simulink model "SCARA_Ass5_Script_Visual"  (Simulink 7.4)
settings: Solver=FixedStepDiscrete  StartTime=0.0  StopTime=inf  FixedStep=0.00001  RelTol=1e-3
libraries: vrlib x1
settings Model: Creator=Mengchen  LastModifiedBy=t6z8
settings OptimizationCC: ExpressionDepthLimit=128  InitFltsAndDblsToZero=on
settings DebuggingCC: AlgebraicLoopMsg=error  SaveWithParameterizedLinksMsg=none  StateNameClashWarn=none  StrictBusMsg=ErrorLevel1
settings HardwareCC: TargetEndianess=LittleEndian  TargetHWDeviceType=MATLAB Host
settings RTWCC: ProcessScript=grt_make_rtw_hook  CustomHeaderCode="#include \"haptics.h\""  CustomInclude="\"C:\\Program Files\\novint\\HDAL_SDK_1.1.0_Beta\\include\""  TargetLang=C++
settings CodeAppCC: CustomSymbolStrType=$N$R$M_T

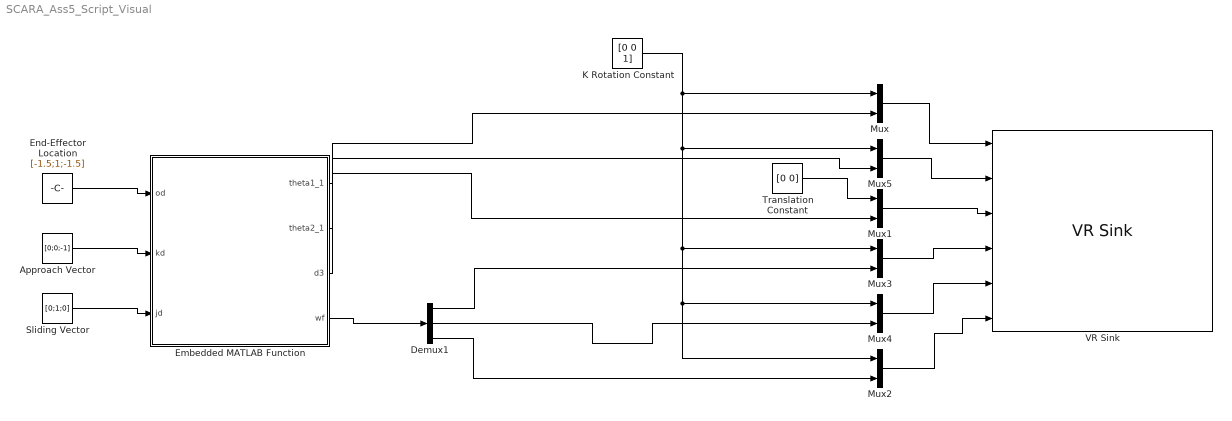
== system SCARA_Ass5_Script_Visual ==
  Approach Vector : Constant  Value=[0;0;-1]
  Demux1 : Demux  Outputs=3
  Embedded MATLAB Function : Stateflow chart
  End-Effector Location : Constant  Value=[-1.5;1;-1.5]
  K Rotation Constant : Constant  Value=[0 0 1]
  Mux{,1..5} (6 alike) : Mux  Inputs=2
  Sliding Vector : Constant  Value=[0;1;0]
  Translation Constant : Constant  Value=[0 0]
  VR Sink : vrlib/VR Sink  InstantiateOnLoad=on  SampleTime=-1  ViewEnable=on  RemoteChange=off  RemoteView=on  FieldsWritten=Link_0_Rotation.rotation.4.1.double#Link_1_Rotation.rotation.4.1.double#Link_2_Translation.translation.3.1.double#Link_3_Rotation.rotation.4.1.double#Link_4_Rotation.rotation.4.1.double#Link_5_Rotation.rotation.4.1.double  WorldFileName=SCARAWORLD.WRL  AutoView=off  VideoDimensions=[]  FigureProperties="{'Position', 'Name', 'Viewpoint', 'CameraBound', 'CameraDirection', 'CameraPosition', 'CameraUpVector', 'ZoomFactor', 'Antialiasing', 'Headlight', 'Lighting', 'NavPanel', 'StatusBar', 'ToolBar', 'Textures', 'Transparency', 'Wireframe', 'NavZones', 'NavMode', 'NavSpeed', 'Record2DCompressMethod', 'Record2DCompressQuality', 'Record2D', 'Record2DFileName', 'Record2DFPS'; [7.7000000000000000e+002  2.2200000000000000e+002  5.7600000000000000e+002  3.8000000000000000e+002], '', 'Viewpoint', 'on', [0.0000000000000000e+000  0.0000000000000000e+000 -1.0000000000000000e+000], [0.0000000000000000e+000  0.0000000000000000e+000  0.0000000000000000e+000], [0.0000000000000000e+000  1.0000000000000000e+000  0.0000000000000000e+000], [1.0000000000000000e+000], 'off', 'on', 'on', 'halfbar', 'on', 'on', 'on', 'on', 'off', 'off', 'fly', 'normal', 'auto', [7.5000000000000000e+001], 'off', '%f_anim_%n.avi', [1.5000000000000000e+001]}"
  wires:
  K Rotation Constant/1 -> Mux/1, Mux3/1, Mux4/1, Mux2/1, Mux5/1
  Mux/1 -> VR Sink/1
  Mux1/1 -> VR Sink/3
  Translation Constant/1 -> Mux1/1
  Mux3/1 -> VR Sink/4
  Mux4/1 -> VR Sink/5
  Mux2/1 -> VR Sink/6
  Mux5/1 -> VR Sink/2
  Embedded MATLAB Function/1(theta1_1) -> Mux/2
  Embedded MATLAB Function/2(theta2_1) -> Mux5/2
  Embedded MATLAB Function/3(d3) -> Mux1/2
  Demux1/1 -> Mux3/2
  Demux1/2 -> Mux4/2
  Demux1/3 -> Mux2/2
  Embedded MATLAB Function/4(wf) -> Demux1/1
  Approach Vector/1 -> Embedded MATLAB Function/2(kd)
  End-Effector Location/1 -> Embedded MATLAB Function/1(od)
  Sliding Vector/1 -> Embedded MATLAB Function/3(jd)

== matlab function Embedded MATLAB Function ==
  data: od input double; theta1_1 output double; theta2_1 output double; d3 output double; kd input double; jd input double; wf output double
function [theta1_1, theta2_1, d3, wf] = hw5_inverse_function(od, kd, jd)

l1 = 1;
l2 = 1;
l3 = 0.5;
l6 = 0.2;

i = [1; 0; 0];
j = [0; 1; 0];
k = [0; 0; 1];

kx = [0 0 0;
      0 0 -1;
      0 1 0];

o0 = [0; 0; 0];
C0 = eye(3);

coord0 = [C0 o0;
          zeros(1,3) 1];

% Ask for o6, approach vector and sliding vector
%od = input('Enter od ([od_i; od_j; od_k]): ');
%kd = input('Enter approach vector (kd) ([kd_i; kd_j; kd_k]): ');
%jd = input('Enter sliding vector (jd) ([jd_i; jd_j; jd_k]): ');
id = -cross(kd, jd);

Cd = [id jd kd];

% Calculate wrist center

o3 = od - Cd*l6*k;

o2 = o3;

o2(3) = l3+l6;

d3 = o2(3) - o3(3) - l3;

% Solve inverse arm kinematics
% see Slide 1 of Inverse Kinematics slides
u = o2 - o0;
l = sqrt(u(1)*u(1) + u(2)*u(2));

theta2_1 = pi - acos((-l^2 + l1^2 + l2^2)/(2*l1*l2));

alpha = atan(-u(1)/u(2));

% the atan always returns a value between -pi/2 and pi/2,
% so you have to check if the point you want to reach is in the left half
if u(2) < 0
    alpha = alpha + pi;
end

beta = acos((-l2^2 + l1^2 + l^2)/(2*l1*l));

theta1_1 = alpha - beta;

% other solution

%theta1_2 = alpha + beta;
%theta2_2 = -theta2_1;

% there are infinte solutions for theta1 if the gripper is supposed
% to be at the origin ([0; 0; 0])
if isnan(u(1)/u(2))
    %disp('Infinite solutions for theta1, just displaying one with theta1 = 0');
    theta1_1 = 0;
    theta2_1 = pi;
    
    %theta1_2 = 0;
    %theta2_2 = pi;
end

%a1 = [ (theta1_1* (pi / 180)), (theta2_1* (pi / 180)), d3];
%a1 = [a1;a1];
%a2 = [ theta1_2, theta2_2, d3];
%a2 = [a2;a2];

% Get wrist base frame by direct kinematics
coord3_1 = solve_arm_forward(coord0, theta1_1, theta2_1, d3);
%coord3_2 = solve_arm_forward(coord0, theta1_2, theta2_2, d3);

w1 = solve_wrist_inverse(coord3_1,  od, kd, jd);
wf=w1(2,:);
%w2 = solve_wrist_inverse(coord3_2,  od, kd, jd);

%result = [ a1 w1; a2 w2]
